simulink library "myLibrary"  (R2023b)
settings: Solver=VariableStepAuto  StartTime=0.0  StopTime=10.0  RelTol=1e-3
undefined symbols (not defined in the file): Cac_n1, ctrl1, Da, Discrete, dtha, ee_sli_rtmsupport, FA, gcbh, Ha, Ini, init_DCline, init_IPC, init_line, init_load, init_SG, init_shunt, init_TH, init_trafo, init_VSC, initMachineBlocks, Ka, Lf, Llkd_pu, Llkq1_pu, magnitude, NET, P, plots_step, q0, Rac_n1, Radd, Rkd_pu, Rkq1_pu, Rload_add, sim_config, sps_rtmsupport, spsSteamTurbineModel, T_DC_NET, T_global, T_IPC, T_load, T_NET, T_SG, T_shunt, T_STATCOM, T_TH, T_trafo, T_VSC, Ts, tstep, Udiff_a, V1
libraries: spsSeriesRLCBranchLib x105, eeGeneralControl x72, $bdroot x70, spsCurrentMeasurementLib x48, spsParallelRLCBranchLib x39, spsVoltageMeasurementLib x33, spsControlledVoltageSourceLib x27, spsFirstOrderFilterLib x16, dspsigops x6, spsThreePhaseVIMeasurementLib x5, spsPLL3phLib x4, spsThreePhaseBreakerLib x3
(part 1 of 12)
settings Model: Creator=CITCEA  LastModifiedBy=Josep
settings DebuggingCC: UnconnectedInputMsg=warning  UnconnectedOutputMsg=warning  UnconnectedLineMsg=warning
settings ModelReferenceCC: EnableRefExpFcnMdlSchedulingChecks=on
settings RTWCC: DLArmComputeVersion=19.05

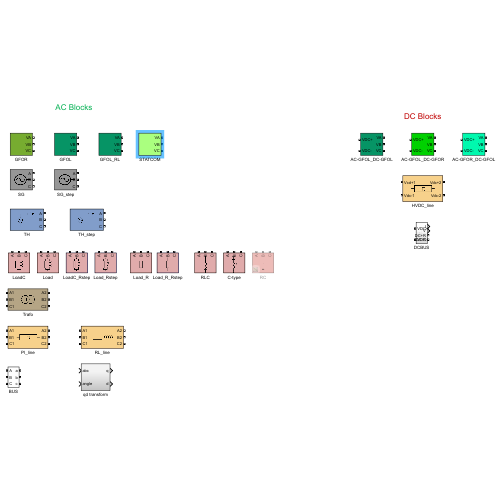
[thumbnail: Simulink's stored preview of the top-level diagram]
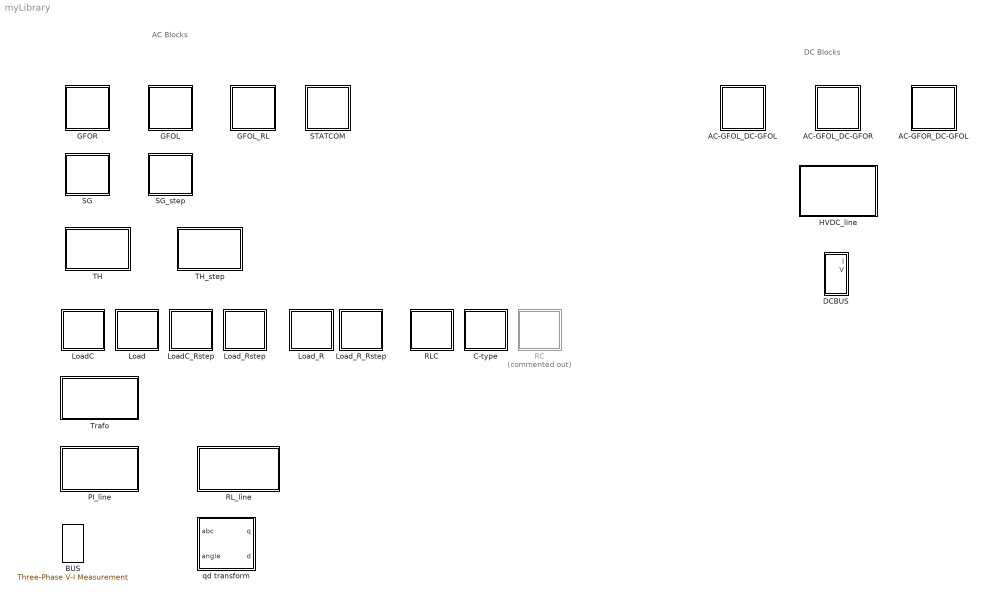
== system myLibrary ==
  note: DC Blocks
  note: AC Blocks
  AC-GFOL_DC-GFOL : Subsystem  mask{T_IPC_global=T_IPC, initIPC_global=init_IPC, num=1}
      mask prompts: T_IPC_global "T_IPC"; initIPC_global "init_IPC"
      mask init:
      | T_IPC = T_IPC_global(num,:);
      | initIPC = initIPC_global{num};
      | 
      | %set_param([gcb '/Control/Goto_w'],'GotoTag',['w_GFOL' num2str(num)])
      | %set_param([gcb '/Control/From_w'],'GotoTag',['w_GFOL' num2str(num)])
  AC-GFOL_DC-GFOR : Subsystem  mask{T_IPC_global=T_IPC, initIPC_global=init_IPC, num=1}
      mask prompts: T_IPC_global "T_IPC"; initIPC_global "init_IPC"
      mask init:
      | T_IPC = T_IPC_global(num,:);
      | initIPC = initIPC_global{num};
      | 
      | %set_param([gcb '/Control/Goto_w'],'GotoTag',['w_GFOL' num2str(num)])
      | %set_param([gcb '/Control/From_w'],'GotoTag',['w_GFOL' num2str(num)])
  AC-GFOR_DC-GFOL : Subsystem  mask{T_IPC_global=T_IPC, initIPC_global=init_IPC, num=1}
      mask prompts: T_IPC_global "T_IPC"; initIPC_global "init_IPC"
      mask init:
      | T_IPC = T_IPC_global(num,:);
      | initIPC = initIPC_global{num};
      | 
      | %set_param([gcb '/Control/Goto_w'],'GotoTag',['w_GFOL' num2str(num)])
      | %set_param([gcb '/Control/From_w'],'GotoTag',['w_GFOL' num2str(num)])
  BUS : spsThreePhaseVIMeasurementLib/Three-Phase V-I Measurement  VoltageMeasurement=phase-to-phase  SetLabelV=on  LabelV=V  Vpu=off  VpuLL=off  CurrentMeasurement=yes  SetLabelI=on  LabelI=I  Ipu=off  Pbase=100e6  Vbase=500e3  OutputType=Complex  PhasorSimulation=off  PSBequivalent=0
  C-type : Subsystem  mask{T_shunt_global=T_shunt, initShunt_global=init_shunt, num=1}
      mask prompts: T_shunt_global "T_shunt"; initShunt_global "init_shunt"
      mask init:
      | T = T_shunt_global(num,:);
      | ini = initShunt_global{num};
      mask Display:
      | % Use specified image as mask icon
      | image('C-type.png')
  DCBUS : Subsystem
  GFOL : Subsystem  mask{T_VSC_global=T_VSC, initVSC_global=init_VSC, num=1}
      mask prompts: T_VSC_global "T_VSC"; initVSC_global "init_VSC"
      mask init:
      | T_VSC = T_VSC_global(num,:);
      | initVSC = initVSC_global{num};
      | 
      | set_param([gcb '/Control/Goto_w'],'GotoTag',['w_GFOL' num2str(num)])
      | set_param([gcb '/Control/From_w'],'GotoTag',['w_GFOL' num2str(num)])
  GFOL_RL : Subsystem  mask{T_VSC_global=T_VSC, initVSC_global=init_VSC, num=1}
      mask prompts: T_VSC_global "T_VSC"; initVSC_global "init_VSC"
      mask init:
      | T_VSC = T_VSC_global(num,:);
      | initVSC = initVSC_global{num};
      | 
      | set_param([gcb '/Control/Goto_w'],'GotoTag',['w_GFOL' num2str(num)])
      | set_param([gcb '/Control/From_w'],'GotoTag',['w_GFOL' num2str(num)])
  GFOR : Subsystem  mask{T_VSC_global=T_VSC, initVSC_global=init_VSC, num=1}
      mask prompts: T_VSC_global "T_VSC"; initVSC_global "init_VSC"
      mask init:
      | T_VSC = T_VSC_global(num,:);
      | initVSC = initVSC_global{num};
      | 
      | set_param([gcb '/Control/Goto_theta'],'GotoTag',['theta_GFOR' num2str(num)])
      | set_param([gcb '/Control/PLL/Goto_w'],'GotoTag',['w_GFOR' num2str(num)])
  HVDC_line : Subsystem  mask{T_HVDC_line_global=T_DC_NET, initDCLine_global=init_DCline, num=1}
      mask prompts: T_HVDC_line_global "T_DC_line"; initDCLine_global "init_DCline"
      mask init:
      | T = T_HVDC_line_global(num,:);
      | ini = initDCLine_global{num};
      mask Display:
      | % Use specified image as mask icon
      | image('PI.png')
  Load : Subsystem  mask{T_load_global=T_load, initLoad_global=init_load, num=1}
      mask prompts: T_load_global "T_load"; initLoad_global "init_load"
      mask init:
      | T = T_load_global(num,:);
      | ini = initLoad_global{num};
      mask Display:
      | % Use specified image as mask icon
      | image('load.png')
  LoadC : Subsystem  mask{T_load_global=T_load, initLoad_global=init_load, num=1}
      mask prompts: T_load_global "T_load"; initLoad_global "init_load"
      mask init:
      | T = T_load_global(num,:);
      | ini = initLoad_global{num};
      mask Display:
      | % Use specified image as mask icon
      | image('load.png')
  LoadC_Rstep : Subsystem  mask{T_load_global=T_load, initLoad_global=init_load, num=1, tstep=tstep, Radd=Radd}
      mask prompts: T_load_global "T_load"; initLoad_global "init_load"
      mask init:
      | T = T_load_global(num,:);
      | ini = initLoad_global{num};
      mask Display:
      | % Use specified image as mask icon
      | image('load.png')
  Load_R : Subsystem  mask{T_load_global=T_load, num=1}
      mask prompts: T_load_global "T_load"
      mask init:
      | T = T_load_global(num,:);
      mask Display:
      | % Use specified image as mask icon
      | image('load_R.png')
  Load_R_Rstep : Subsystem  mask{T_load_global=T_load, num=1, tstep=tstep, Radd=Radd}
      mask prompts: T_load_global "T_load"
      mask init:
      | T = T_load_global(num,:);
      mask Display:
      | % Use specified image as mask icon
      | image('load_R.png')
  Load_Rstep : Subsystem  mask{T_load_global=T_load, initLoad_global=init_load, num=1, tstep=tstep, Radd=Radd}
      mask prompts: T_load_global "T_load"; initLoad_global "init_load"
      mask init:
      | T = T_load_global(num,:);
      | ini = initLoad_global{num};
      mask Display:
      | % Use specified image as mask icon
      | image('load.png')
  PI_line : Subsystem  mask{T_line_global=T_NET, initLine_global=init_line, num=1, set_C0=ones(1,6), set_iL0=0}
      mask prompts: T_line_global "T_line"; initLine_global "init_line"; set_C0 "init_cap"; set_iL0 "init_ind"
      mask init:
      | T = T_line_global(num,:);
      | ini = initLine_global{num};
      | set_C00 = set_C0(1,1);
      | set_C01 = set_C0(1,2);
      | set_C02 = set_C0(1,3);
      | set_C03 = set_C0(1,4);
      | set_C04 = set_C0(1,5);
      | set_C05 = set_C0(1,6);
      | set_param([gcb '/Series RLC Branch'],'Setx0',set_C00)
      | set_param([gcb '/Series RLC Branch1'],'Setx0',set_C01)
      | set_param([gcb '/Series RLC Branch2'],'Setx0',set_C02)
      | set_param([gcb '/Series RLC Branch3'],'Setx0',set_C03)
      | set_param([gcb '/Series RLC Branch4'],'Setx0',set_C04)
      | set_param([gcb '/Series RLC Branch5'],'Setx0',set_C05)
      | set_param([gcb '/Series RLC Branch6'],'SetiL0',set_iL0)
      mask Display:
      | % Use specified image as mask icon
      | image('PI.png')
  RC : Subsystem  Commented=on  mask{T_shunt_global=T_shunt, initShunt_global=init_shunt, num=1}
      mask prompts: T_shunt_global "T_shunt"; initShunt_global "init_shunt"
      mask init:
      | T = T_shunt_global(num,:);
      | ini = initShunt_global{num};
      mask Display:
      | % Use specified image as mask icon
      | image('RC.png')
  RLC : Subsystem  mask{T_shunt_global=T_shunt, initShunt_global=init_shunt, num=1}
      mask prompts: T_shunt_global "T_shunt"; initShunt_global "init_shunt"
      mask init:
      | T = T_shunt_global(num,:);
      | ini = initShunt_global{num};
      mask Display:
      | % Use specified image as mask icon
      | image('RLC.png')
  RL_line : Subsystem  mask{T_line_global=T_NET, initLine_global=init_line, num=1}
      mask prompts: T_line_global "T_line"; initLine_global "init_line"
      mask init:
      | T = T_line_global(num,:);
      | ini = initLine_global{num};
      mask Display:
      | % Use specified image as mask icon
      | image('RL.png')
  SG : Subsystem  mask{num=1, init_SG_global=init_SG, initMachineBlocks=initMachineBlocks, T_SG_global=T_SG}
      mask prompts: init_SG_global "init_SG"; initMachineBlocks "initMachine"; T_SG_global "T_SG"
      mask init:
      | initSG = init_SG_global{num};
      | T_SG = T_SG_global(num,:);
      | SGnum = num;
      | 
      | T_SG.exc = T_SG.exc{:};
      | T_SG.mech = T_SG.mech{:};
      | T_SG.PSS = T_SG.PSS{:};
      | 
      | 
      | switch T_SG.pss{:}
      |     case '2A'
      |         hasPSS = 1;
      |         set_param([gcb '/Exciter/PSS 2A'],'commented', 'off')
      |     case 'no'
      |         hasPSS = 0;
      |         set_param([gcb '/Exciter/PSS 2A'],'commented', 'on')
      | end
      | 
      | switch T_SG.govturb{:}
      |     case 'IEEEG1'
      |         selectGovturb= 1;
      |         set_param([gcb '/Governor-Turbine/IEEEG1'],'commented', 'off')
      |         set_param([gcb '/Governor-Turbine/Steam Turbine and Governor'],'commented', 'on')
      |     case 'TANDEM-SINGLE'
      |         selectGovturb= 2;
      |         T_SG.genType = 0;
      |         set_param([gcb '/Governor-Turbine/IEEEG1'],'commented', 'on')
      |         set_param([gcb '/Governor-Turbine/Steam Turbine and Governor'],'commented', 'off')
      |     case 'TANDEM-MULTI'
      |         selectGovturb= 2;
      |         T_SG.genType = 1;
      |         set_param([gcb '/Governor-Turbine/IEEEG1'],'commented', 'on')
      |         set_param([gcb '/Governor-Turbine/Steam Turbine and Governor'],'commented', 'off')
      |     case 'no'
      |         selectGovturb= 3;
      |         set_param([gcb '/Governor-Turbine/IEEEG1'],'commented', 'on')
      |         set_param([gcb '/Governor-Turbine/Steam Turbine and Governor'],'commented', 'on')
      | end
      | 
      | switch T_SG.exciter{:} 
      |     case 'AC4A'
      |         selectExciter = 1;
      |         set_param([gcb '/Exciter/Exciter AC4A'],'commented', 'off')
      |         set_param([gcb '/Exciter/Exciter ST4B'],'commented', 'on')
      |         set_param([gcb '/Exciter/Exciter ST1'],'commented', 'on')
      |     case 'ST4B'
      |         selectExciter = 2;
      |         set_param([gcb '/Exciter/Exciter AC4A'],'commented', 'on')
      |         set_param([gcb '/Exciter/Exciter ST4B'],'commented', 'off')
      |         set_param([gcb '/Exciter/Exciter ST1'],'commented', 'on')
      |     case 'ST1'
      |         selectExciter = 3;
      |         set_param([gcb '/Exciter/Exciter AC4A'],'commented', 'on')
      |         set_param([gcb '/Exciter/Exciter ST4B'],'commented', 'on')
      |         set_param([gcb '/Exciter/Exciter ST1'],'commented', 'off')
      |     case 'no'
      |         selectExciter = 4;
      |         set_param([gcb '/Exciter/Exciter AC4A'],'commented', 'on')
      |         set_param([gcb '/Exciter/Exciter ST4B'],'commented', 'on')
      |         set_param([gcb '/Exciter/Exciter ST1'],'commented', 'on')
      | end
      | 
      | set_param([gcb '/Goto_theta'],'GotoTag',['theta_SG' num2str(SGnum)])
      | set_param([gcb '/Goto_w'],'GotoTag',['w_SG' num2str(SGnum)])
      mask Display:
      | % Use specified image as mask icon
      | image('SG.png')
  SG_step : Subsystem  mask{num=1, init_SG_global=init_SG, initMachineBlocks=initMachineBlocks, T_SG_global=T_SG, step_var=Pref, tstep=sim_config.tstep}
      mask prompts: init_SG_global "init_SG"; initMachineBlocks "initMachine"; T_SG_global "T_SG"
      mask init:
      | initSG = init_SG_global{num};
      | T_SG = T_SG_global(num,:);
      | SGnum = num;
      | 
      | T_SG.exc = T_SG.exc{:};
      | T_SG.mech = T_SG.mech{:};
      | T_SG.PSS = T_SG.PSS{:};
      | 
      | 
      | switch T_SG.pss{:}
      |     case '2A'
      |         hasPSS = 1;
      |         set_param([gcb '/Exciter/PSS 2A'],'commented', 'off')
      |     case 'no'
      |         hasPSS = 0;
      |         set_param([gcb '/Exciter/PSS 2A'],'commented', 'on')
      | end
      | 
      | switch T_SG.govturb{:}
      |     case 'IEEEG1'
      |         selectGovturb= 1;
      |         set_param([gcb '/Governor-Turbine/IEEEG1'],'commented', 'off')
      |         set_param([gcb '/Governor-Turbine/Steam Turbine and Governor'],'commented', 'on')
      |     case 'TANDEM-SINGLE'
      |         selectGovturb= 2;
      |         T_SG.genType = 0;
      |         set_param([gcb '/Governor-Turbine/IEEEG1'],'commented', 'on')
      |         set_param([gcb '/Governor-Turbine/Steam Turbine and Governor'],'commented', 'off')
      |     case 'TANDEM-MULTI'
      |         selectGovturb= 2;
      |         T_SG.genType = 1;
      |         set_param([gcb '/Governor-Turbine/IEEEG1'],'commented', 'on')
      |         set_param([gcb '/Governor-Turbine/Steam Turbine and Governor'],'commented', 'off')
      |     case 'no'
      |         selectGovturb= 3;
      |         set_param([gcb '/Governor-Turbine/IEEEG1'],'commented', 'on')
      |         set_param([gcb '/Governor-Turbine/Steam Turbine and Governor'],'commented', 'on')
      | end
      | 
      | switch T_SG.exciter{:} 
      |     case 'AC4A'
      |         selectExciter = 1;
      |         set_param([gcb '/Exciter/Exciter AC4A'],'commented', 'off')
      |         set_param([gcb '/Exciter/Exciter ST4B'],'commented', 'on')
      |         set_param([gcb '/Exciter/Exciter ST1'],'commented', 'on')
      |     case 'ST4B'
      |         selectExciter = 2;
      |         set_param([gcb '/Exciter/Exciter AC4A'],'commented', 'on')
      |         set_param([gcb '/Exciter/Exciter ST4B'],'commented', 'off')
      |         set_param([gcb '/Exciter/Exciter ST1'],'commented', 'on')
      |     case 'ST1'
      |         selectExciter = 3;
      |         set_param([gcb '/Exciter/Exciter AC4A'],'commented', 'on')
      |         set_param([gcb '/Exciter/Exciter ST4B'],'commented', 'on')
      |         set_param([gcb '/Exciter/Exciter ST1'],'commented', 'off')
      |     case 'no'
      |         selectExciter = 4;
      |         set_param([gcb '/Exciter/Exciter AC4A'],'commented', 'on')
      |         set_param([gcb '/Exciter/Exciter ST4B'],'commented', 'on')
      |         set_param([gcb '/Exciter/Exciter ST1'],'commented', 'on')
      | end
      | 
      | set_param([gcb '/Goto_theta'],'GotoTag',['theta_SG' num2str(SGnum)])
      | set_param([gcb '/Goto_w'],'GotoTag',['w_SG' num2str(SGnum)])
      | 
      | switch step_var
      |     case 'Pref'
      |         tstep_P = tstep;
      |         tstep_V = 1e3;
      |     case 'Vref'
      |         tstep_P = 1e3;
      |         tstep_V = tstep;
      | end
      mask TypeOptions step_var: Pref | Vref
      mask Display:
      | % Use specified image as mask icon
      | image('SG.png')
  STATCOM : Subsystem  mask{T_VSC_global=T_VSC, initVSC_global=init_VSC, num=1}
      mask prompts: T_VSC_global "T_VSC"; initVSC_global "init_VSC"
      mask init:
      | T_VSC = T_VSC_global(num,:);
      | initVSC = initVSC_global{num};
      | 
      | switch T_VSC.POD{:}
      |     case 'Yes'
      |         POD = 1;
      |         set_param([gcb '/Control/POD'],'commented', 'off')
      |         set_param([gcb '/Control/From34'],'commented', 'off')
      |         set_param([gcb '/Control/From35'],'commented', 'off')
      |         set_param([gcb '/Control/From36'],'commented', 'off')
      |         set_param([gcb '/Control/From37'],'commented', 'off')
      |     case 'No'
      |         POD = 2;
      |         set_param([gcb '/Control/POD'],'commented', 'on')
      |         set_param([gcb '/Control/From34'],'commented', 'on')
      |         set_param([gcb '/Control/From35'],'commented', 'on')
      |         set_param([gcb '/Control/From36'],'commented', 'on')
      |         set_param([gcb '/Control/From37'],'commented', 'on')
      | end
      | 
      | 
      | 
      | set_param([gcb '/Control/Goto_w'],'GotoTag',['w_STATCOM' num2str(num)])
  TH : Subsystem  mask{T_TH_global=T_TH, initTH_global=init_TH, num=1}
      mask prompts: T_TH_global "T_TH"; initTH_global "init_TH"
      mask init:
      | T = T_TH_global(num,:);
      | ini = initTH_global{num};
      mask Display:
      | port_label('rconn', 1, 'A')
      | port_label('rconn', 2, 'B')
      | port_label('rconn', 3, 'C')
      | 
      | % Use specified image as mask icon
      | image('TH.png')
  TH_step : Subsystem  mask{T_TH_global=T_TH, initTH_global=init_TH, num=1, tstep=tstep, V1=V1}
      mask prompts: T_TH_global "T_TH"; initTH_global "init_TH"
      mask init:
      | T = T_TH_global(num,:);
      | ini = initTH_global{num};
      mask Display:
      | port_label('rconn', 1, 'A')
      | port_label('rconn', 2, 'B')
      | port_label('rconn', 3, 'C')
      | 
      | % Use specified image as mask icon
      | image('TH.png')
  Trafo : Subsystem  mask{T_trafo_global=T_trafo, initTrafo_global=init_trafo, num=3}
      mask prompts: T_trafo_global "T_trafo"; initTrafo_global "init_trafo"
      mask init:
      | T = T_trafo_global(num,:);
      | ini = initTrafo_global{num};
      mask Display:
      | % Use specified image as mask icon
      | image('trafo.png')
  qd transform : Subsystem

== system myLibrary/AC-GFOL_DC-GFOL ==
  Constant1 : Constant  Value=[ 2/3 1/3; -1/3 1/3 ; -1/3 -2/3]
  Control Pac2 : Subsystem
      settings: PortSchema="{\"entries\":[{\"content\":{\"sides\":[{\"content\":{},\"type\":\"ConnectorPlacement.EquallySpacedRectSide\",\"uuid\":\"681c0b5f-022d-4b6d-8fe2-73940743a76e\"},{\"content\":{\"side\":\"RIGHT\"},\"type\":\"ConnectorPlacement.EquallySpacedRectSide\",\"uuid\":\"e9b400c8-e13f-4caf-91a1-f348979675fd\"},{\"content\":{\"connectorIds\":[\"Out1\"],\"side\":\"TOP\"},\"type\":\"ConnectorPlacement.EquallySpacedRectSide\",\"uuid\":\"348007cb-ce67-4c45-ad7b-36ba89db6185\"},{\"content\":{\"connectorIds\":[\"In1\",\"In2\",\"In3\",\"In4\",\"In5\",\"In6\"],\"side\":\"BOTTOM\"},\"type\":\"ConnectorPlacement.EquallySpacedRectSide\",\"uuid\":\"fd6a847a-5d69-44cd-a0d1-495126761350\"}]},\"type\":\"ConnectorPlacement.EquallySpacedConnector\",\"uuid\":\"d16b8cae-5ced-4c76-a87e-983e154fb48f\"}],\"packageUris\":[\"http://schema.mathworks.com/mf0/Connector/R2020b\"],\"version\":\"1.0\"}"
  Is_l2g1 : Gain  Gain=1/T_IPC.Ibpu_l2g
  Is_l2g2 : Gain  Gain=1/T_IPC.Ibpu_l2g
  Is_l2g3 : Gain  Gain=1/T_IPC.Ibpu_l2g
  MMC1 : Subsystem
  Mesura Ulina12 : spsVoltageMeasurementLib/Voltage Measurement  PhasorSimulation=off  OutputType=Complex  PSBequivalent=0
  Mux1 : Mux  Inputs=2
  Product1 : Product  Multiplication=Matrix(*)
  Scope : Scope
  Scope1 : Scope
  U_g2l1 : Gain  Gain=1/T_IPC.Vbpu_l2g
  U_g2l2 : Gain  Gain=1/T_IPC.Vbpu_l2g
  U_g2l3 : Gain  Gain=1/T_IPC.Vbpu_l2g
  Vdiff_l2g1 : Gain  Gain=T_IPC.Vbpu_l2g
  Voltage Measurement2 : spsVoltageMeasurementLib/Voltage Measurement  PhasorSimulation=off  OutputType=Complex  PSBequivalent=0
  Voltage Measurement3 : spsVoltageMeasurementLib/Voltage Measurement  PhasorSimulation=off  OutputType=Complex  PSBequivalent=0
  VA : PMIOPort  Side=Right
  VB : PMIOPort  Port=2  Side=Right
  VC : PMIOPort  Port=3  Side=Right
  VDC+ : PMIOPort  Port=4  Side=Left
  VDC- : PMIOPort  Port=5  Side=Left
  wires:
  Voltage Measurement3/1 -> Mux1/2
  Mux1/1 -> Product1/2
  Constant1/1 -> Product1/1
  MMC1/4(Vs) -> U_g2l2/1
  Product1/1 -> Scope1/1, U_g2l1/1
  Control Pac2/1(Vdiff-sum) -> Vdiff_l2g1/1
  Mesura Ulina12/1 -> U_g2l3/1, Scope/1
  MMC1/2(Iu) -> Is_l2g2/1
  MMC1/1(Is) -> Is_l2g3/1
  MMC1/3(Il) -> Is_l2g1/1
  Voltage Measurement2/1 -> Mux1/1
  Vdiff_l2g1/1 -> MMC1/1(Vdiff,sum)
  U_g2l1/1 -> Control Pac2/1(U)
  U_g2l2/1 -> Control Pac2/3(Vs)
  U_g2l3/1 -> Control Pac2/2(Vdc2)
  Is_l2g1/1 -> Control Pac2/4(Il)
  Is_l2g2/1 -> Control Pac2/5(Iu)
  Is_l2g3/1 -> Control Pac2/6(Iss)
  connections:
  Voltage Measurement3/LConn1 -- MMC1/LConn2 -- Voltage Measurement2/LConn2 -- VB/RConn1
  VDC-/RConn1 -- MMC1/RConn2 -- Mesura Ulina12/LConn2
  Voltage Measurement2/LConn1 -- MMC1/LConn1 -- VA/RConn1
  VDC+/RConn1 -- MMC1/RConn1 -- Mesura Ulina12/LConn1
  VC/RConn1 -- MMC1/LConn3 -- Voltage Measurement3/LConn2

== system myLibrary/AC-GFOL_DC-GFOR ==
  Constant1 : Constant  Value=[ 2/3 1/3; -1/3 1/3 ; -1/3 -2/3]
  Control Pac2 : Subsystem
      settings: PortSchema="{\"entries\":[{\"content\":{\"sides\":[{\"content\":{},\"type\":\"ConnectorPlacement.EquallySpacedRectSide\",\"uuid\":\"681c0b5f-022d-4b6d-8fe2-73940743a76e\"},{\"content\":{\"side\":\"RIGHT\"},\"type\":\"ConnectorPlacement.EquallySpacedRectSide\",\"uuid\":\"e9b400c8-e13f-4caf-91a1-f348979675fd\"},{\"content\":{\"connectorIds\":[\"Out1\"],\"side\":\"TOP\"},\"type\":\"ConnectorPlacement.EquallySpacedRectSide\",\"uuid\":\"348007cb-ce67-4c45-ad7b-36ba89db6185\"},{\"content\":{\"connectorIds\":[\"In1\",\"In2\",\"In3\",\"In4\",\"In5\",\"In6\"],\"side\":\"BOTTOM\"},\"type\":\"ConnectorPlacement.EquallySpacedRectSide\",\"uuid\":\"fd6a847a-5d69-44cd-a0d1-495126761350\"}]},\"type\":\"ConnectorPlacement.EquallySpacedConnector\",\"uuid\":\"d16b8cae-5ced-4c76-a87e-983e154fb48f\"}],\"packageUris\":[\"http://schema.mathworks.com/mf0/Connector/R2020b\"],\"version\":\"1.0\"}"
  Is_l2g1 : Gain  Gain=1/T_IPC.Ibpu_l2g
  Is_l2g2 : Gain  Gain=1/T_IPC.Ibpu_l2g
  Is_l2g3 : Gain  Gain=1/T_IPC.Ibpu_l2g
  MMC1 : Subsystem
  Mesura Ulina12 : spsVoltageMeasurementLib/Voltage Measurement  PhasorSimulation=off  OutputType=Complex  PSBequivalent=0
  Mux1 : Mux  Inputs=2
  Product1 : Product  Multiplication=Matrix(*)
  Scope : Scope
  Scope1 : Scope
  U_g2l1 : Gain  Gain=1/T_IPC.Vbpu_l2g
  U_g2l2 : Gain  Gain=1/T_IPC.Vbpu_l2g
  U_g2l3 : Gain  Gain=1/T_IPC.Vbpu_l2g
  Vdiff_l2g1 : Gain  Gain=T_IPC.Vbpu_l2g
  Voltage Measurement2 : spsVoltageMeasurementLib/Voltage Measurement  PhasorSimulation=off  OutputType=Complex  PSBequivalent=0
  Voltage Measurement3 : spsVoltageMeasurementLib/Voltage Measurement  PhasorSimulation=off  OutputType=Complex  PSBequivalent=0
  VA : PMIOPort  Side=Right
  VB : PMIOPort  Port=2  Side=Right
  VC : PMIOPort  Port=3  Side=Right
  VDC+ : PMIOPort  Port=4  Side=Left
  VDC- : PMIOPort  Port=5  Side=Left
  wires:
  Voltage Measurement3/1 -> Mux1/2
  Mux1/1 -> Product1/2
  Constant1/1 -> Product1/1
  MMC1/4(Vs) -> U_g2l2/1
  Product1/1 -> Scope1/1, U_g2l1/1
  Control Pac2/1(Vdiff-sum) -> Vdiff_l2g1/1
  Mesura Ulina12/1 -> U_g2l3/1, Scope/1
  MMC1/2(Iu) -> Is_l2g2/1
  MMC1/1(Is) -> Is_l2g3/1
  MMC1/3(Il) -> Is_l2g1/1
  Voltage Measurement2/1 -> Mux1/1
  Vdiff_l2g1/1 -> MMC1/1(Vdiff,sum)
  U_g2l1/1 -> Control Pac2/1(U)
  U_g2l2/1 -> Control Pac2/3(Vs)
  U_g2l3/1 -> Control Pac2/2(Vdc)
  Is_l2g1/1 -> Control Pac2/4(Il)
  Is_l2g2/1 -> Control Pac2/5(Iu)
  Is_l2g3/1 -> Control Pac2/6(Iss)
  connections:
  MMC1/LConn2 -- Voltage Measurement3/LConn1 -- Voltage Measurement2/LConn2 -- VB/RConn1
  MMC1/RConn2 -- VDC-/RConn1 -- Mesura Ulina12/LConn2
  MMC1/LConn1 -- Voltage Measurement2/LConn1 -- VA/RConn1
  VDC+/RConn1 -- Mesura Ulina12/LConn1 -- MMC1/RConn1
  MMC1/LConn3 -- VC/RConn1 -- Voltage Measurement3/LConn2

== system myLibrary/AC-GFOR_DC-GFOL ==
  Constant1 : Constant  Value=[ 2/3 1/3; -1/3 1/3 ; -1/3 -2/3]
  Control Pac2 : Subsystem
      settings: PortSchema="{\"entries\":[{\"content\":{\"sides\":[{\"content\":{},\"type\":\"ConnectorPlacement.EquallySpacedRectSide\",\"uuid\":\"681c0b5f-022d-4b6d-8fe2-73940743a76e\"},{\"content\":{\"side\":\"RIGHT\"},\"type\":\"ConnectorPlacement.EquallySpacedRectSide\",\"uuid\":\"e9b400c8-e13f-4caf-91a1-f348979675fd\"},{\"content\":{\"connectorIds\":[\"Out1\"],\"side\":\"TOP\"},\"type\":\"ConnectorPlacement.EquallySpacedRectSide\",\"uuid\":\"348007cb-ce67-4c45-ad7b-36ba89db6185\"},{\"content\":{\"connectorIds\":[\"In1\",\"In2\",\"In3\",\"In4\",\"In5\",\"In6\"],\"side\":\"BOTTOM\"},\"type\":\"ConnectorPlacement.EquallySpacedRectSide\",\"uuid\":\"fd6a847a-5d69-44cd-a0d1-495126761350\"}]},\"type\":\"ConnectorPlacement.EquallySpacedConnector\",\"uuid\":\"d16b8cae-5ced-4c76-a87e-983e154fb48f\"}],\"packageUris\":[\"http://schema.mathworks.com/mf0/Connector/R2020b\"],\"version\":\"1.0\"}"
  Is_l2g1 : Gain  Gain=1/T_IPC.Ibpu_l2g
  Is_l2g2 : Gain  Gain=1/T_IPC.Ibpu_l2g
  Is_l2g3 : Gain  Gain=1/T_IPC.Ibpu_l2g
  MMC1 : Subsystem
  Mesura Ulina12 : spsVoltageMeasurementLib/Voltage Measurement  PhasorSimulation=off  OutputType=Complex  PSBequivalent=0
  Mux1 : Mux  Inputs=2
  Product1 : Product  Multiplication=Matrix(*)
  Scope : Scope
  U_g2l1 : Gain  Gain=1/T_IPC.Vbpu_l2g
  U_g2l2 : Gain  Gain=1/T_IPC.Vbpu_l2g
  U_g2l3 : Gain  Gain=1/T_IPC.Vbpu_l2g
  Vdiff_l2g1 : Gain  Gain=T_IPC.Vbpu_l2g
  Voltage Measurement2 : spsVoltageMeasurementLib/Voltage Measurement  PhasorSimulation=off  OutputType=Complex  PSBequivalent=0
  Voltage Measurement3 : spsVoltageMeasurementLib/Voltage Measurement  PhasorSimulation=off  OutputType=Complex  PSBequivalent=0
  VA : PMIOPort  Side=Right
  VB : PMIOPort  Port=2  Side=Right
  VC : PMIOPort  Port=3  Side=Right
  VDC+ : PMIOPort  Port=4  Side=Left
  VDC- : PMIOPort  Port=5  Side=Left
  wires:
  Is_l2g3/1 -> Control Pac2/6(Iss)
  Is_l2g2/1 -> Control Pac2/5(Iu)
  Is_l2g1/1 -> Control Pac2/4(Il)
  U_g2l3/1 -> Control Pac2/2(Vdc)
  U_g2l2/1 -> Control Pac2/3(Vs)
  U_g2l1/1 -> Control Pac2/1(U)
  Vdiff_l2g1/1 -> MMC1/1(Vdiff,sum)
  Voltage Measurement2/1 -> Mux1/1
  MMC1/3(Il) -> Is_l2g1/1
  MMC1/1(Is) -> Is_l2g3/1
  MMC1/2(Iu) -> Is_l2g2/1
  Mesura Ulina12/1 -> Scope/1, U_g2l3/1
  Control Pac2/1(Vdiff-sum) -> Vdiff_l2g1/1
  Product1/1 -> U_g2l1/1
  MMC1/4(Vs) -> U_g2l2/1
  Constant1/1 -> Product1/1
  Mux1/1 -> Product1/2
  Voltage Measurement3/1 -> Mux1/2
  connections:
  Voltage Measurement3/LConn2 -- VC/RConn1 -- MMC1/LConn3
  MMC1/RConn1 -- Mesura Ulina12/LConn1 -- VDC+/RConn1
  VA/RConn1 -- Voltage Measurement2/LConn1 -- MMC1/LConn1
  Mesura Ulina12/LConn2 -- VDC-/RConn1 -- MMC1/RConn2
  VB/RConn1 -- Voltage Measurement2/LConn2 -- Voltage Measurement3/LConn1 -- MMC1/LConn2

== system myLibrary/C-type ==
  C1a : spsSeriesRLCBranchLib/Series RLC Branch  LConnTagsString=__new0  RConnTagsString=__new0  BranchType=C  Resistance=T_STATCOM.Rshunt  Inductance=T_STATCOM.Lshunt  SetiL0=off  InitialCurrent=initMMC.iL_a  Capacitance=T.C1*T.Zbpu_l2g  Setx0=on  InitialVoltage=ini.vC1_a  Measurements=Branch voltage
  C1b : spsSeriesRLCBranchLib/Series RLC Branch  LConnTagsString=__new0  RConnTagsString=__new0  BranchType=C  Resistance=T_STATCOM.Rshunt  Inductance=T_STATCOM.Lshunt  SetiL0=off  InitialCurrent=initMMC.iL_a  Capacitance=T.C1*T.Zbpu_l2g  Setx0=on  InitialVoltage=ini.vC1_b  Measurements=Branch voltage
  C1c : spsSeriesRLCBranchLib/Series RLC Branch  LConnTagsString=__new0  RConnTagsString=__new0  BranchType=C  Resistance=T_STATCOM.Rshunt  Inductance=T_STATCOM.Lshunt  SetiL0=off  InitialCurrent=initMMC.iL_a  Capacitance=T.C1*T.Zbpu_l2g  Setx0=on  InitialVoltage=ini.vC1_c  Measurements=Branch voltage
  C2a : spsSeriesRLCBranchLib/Series RLC Branch  LConnTagsString=__new0  RConnTagsString=__new0  BranchType=C  Resistance=T_STATCOM.Rshunt  Inductance=T_STATCOM.L_ctype  SetiL0=on  InitialCurrent=initMMC.iL_ctype_a  Capacitance=T.C2*T.Zbpu_l2g  Setx0=on  InitialVoltage=ini.vC2_a  Measurements=Branch voltage
  C2b : spsSeriesRLCBranchLib/Series RLC Branch  LConnTagsString=__new0  RConnTagsString=__new0  BranchType=C  Resistance=T_STATCOM.Rshunt  Inductance=T_STATCOM.L_ctype  SetiL0=on  InitialCurrent=initMMC.iL_ctype_b  Capacitance=T.C2*T.Zbpu_l2g  Setx0=on  InitialVoltage=ini.vC2_b  Measurements=Branch voltage
  C2c : spsSeriesRLCBranchLib/Series RLC Branch  LConnTagsString=__new0  RConnTagsString=__new0  BranchType=C  Resistance=T_STATCOM.Rshunt  Inductance=T_STATCOM.L_ctype  SetiL0=on  InitialCurrent=initMMC.iL_ctype_c  Capacitance=T.C2*T.Zbpu_l2g  Setx0=on  InitialVoltage=ini.vC2_c  Measurements=Branch voltage
  La : spsSeriesRLCBranchLib/Series RLC Branch  LConnTagsString=__new0  RConnTagsString=__new0  BranchType=L  Resistance=T_STATCOM.Rshunt  Inductance=T.L/T.Zbpu_l2g  SetiL0=on  InitialCurrent=ini.iL_a  Capacitance=T_STATCOM.C2_ctype  Setx0=on  InitialVoltage=initMMC.vc2_a  Measurements=Branch current
  Lb : spsSeriesRLCBranchLib/Series RLC Branch  LConnTagsString=__new0  RConnTagsString=__new0  BranchType=L  Resistance=T_STATCOM.Rshunt  Inductance=T.L/T.Zbpu_l2g  SetiL0=on  InitialCurrent=ini.iL_b  Capacitance=T_STATCOM.C2_ctype  Setx0=on  InitialVoltage=initMMC.vc2_b  Measurements=Branch current
  Lc : spsSeriesRLCBranchLib/Series RLC Branch  LConnTagsString=__new0  RConnTagsString=__new0  BranchType=L  Resistance=T_STATCOM.Rshunt  Inductance=T.L/T.Zbpu_l2g  SetiL0=on  InitialCurrent=ini.iL_c  Capacitance=T_STATCOM.C2_ctype  Setx0=on  InitialVoltage=initMMC.vc2_c  Measurements=Branch current
  Ra : spsSeriesRLCBranchLib/Series RLC Branch  LConnTagsString=__new0  RConnTagsString=__new0  BranchType=R  Resistance=T.R/T.Zbpu_l2g  Inductance=T_STATCOM.Lshunt  SetiL0=off  InitialCurrent=initMMC.iL_a  Capacitance=T_STATCOM.Cshunt  Setx0=off  InitialVoltage=initMMC.vc_a  Measurements=None
  Rb : spsSeriesRLCBranchLib/Series RLC Branch  LConnTagsString=__new0  RConnTagsString=__new0  BranchType=R  Resistance=T.R/T.Zbpu_l2g  Inductance=T_STATCOM.Lshunt  SetiL0=off  InitialCurrent=initMMC.iL_a  Capacitance=T_STATCOM.Cshunt  Setx0=off  InitialVoltage=initMMC.vc_a  Measurements=None
  Rc : spsSeriesRLCBranchLib/Series RLC Branch  LConnTagsString=__new0  RConnTagsString=__new0  BranchType=R  Resistance=T.R/T.Zbpu_l2g  Inductance=T_STATCOM.Lshunt  SetiL0=off  InitialCurrent=initMMC.iL_a  Capacitance=T_STATCOM.Cshunt  Setx0=off  InitialVoltage=initMMC.vc_a  Measurements=None
  A : PMIOPort  Side=Left
  B : PMIOPort  Port=2  Side=Left
  C : PMIOPort  Port=3  Side=Left
  connections:
  C1c/LConn1 -- C/RConn1
  C1b/LConn1 -- B/RConn1
  C1a/LConn1 -- A/RConn1
  C2c/RConn1 -- Rb/RConn1 -- C2a/RConn1 -- Ra/RConn1 -- C2b/RConn1 -- Rc/RConn1
  Rc/LConn1 -- C1c/RConn1 -- Lc/LConn1
  Ra/LConn1 -- C1a/RConn1 -- La/LConn1
  Rb/LConn1 -- Lb/LConn1 -- C1b/RConn1
  C2c/LConn1 -- Lc/RConn1
  C2a/LConn1 -- La/RConn1
  C2b/LConn1 -- Lb/RConn1

== system myLibrary/DCBUS ==
  Current Measurement : spsCurrentMeasurementLib/Current Measurement  PhasorSimulation=off  OutputType=Complex  PSBequivalent=0
  Voltage Measurement : spsVoltageMeasurementLib/Voltage Measurement  PhasorSimulation=off  OutputType=Complex  PSBequivalent=0
  VDC+R : PMIOPort  Side=Right
  VDC-R : PMIOPort  Port=2  Side=Right
  VDC+L : PMIOPort  Port=3  Side=Left
  VDC-L : PMIOPort  Port=4  Side=Left
  I : Outport
  V : Outport  Port=2
  wires:
  Current Measurement/1 -> I/1
  Voltage Measurement/1 -> V/1
  connections:
  Current Measurement/LConn1 -- Voltage Measurement/LConn1 -- VDC+L/RConn1
  Current Measurement/RConn1 -- VDC+R/RConn1
  Voltage Measurement/LConn2 -- VDC-R/RConn1 -- VDC-L/RConn1

== system myLibrary/GFOL ==
  Constant5 : Constant  Value=[ 2/3 1/3; -1/3 1/3 ; -1/3 -2/3]
  Control : Subsystem
      settings: PortSchema="{\"entries\":[{\"content\":{\"sides\":[{\"content\":{},\"type\":\"ConnectorPlacement.EquallySpacedRectSide\",\"uuid\":\"681c0b5f-022d-4b6d-8fe2-73940743a76e\"},{\"content\":{\"side\":\"RIGHT\"},\"type\":\"ConnectorPlacement.EquallySpacedRectSide\",\"uuid\":\"e9b400c8-e13f-4caf-91a1-f348979675fd\"},{\"content\":{\"connectorIds\":[\"In1\",\"Out1\"],\"side\":\"TOP\"},\"type\":\"ConnectorPlacement.EquallySpacedRectSide\",\"uuid\":\"348007cb-ce67-4c45-ad7b-36ba89db6185\"},{\"content\":{\"connectorIds\":[\"In2\",\"In3\"],\"side\":\"BOTTOM\"},\"type\":\"ConnectorPlacement.EquallySpacedRectSide\",\"uuid\":\"fd6a847a-5d69-44cd-a0d1-495126761350\"}]},\"type\":\"ConnectorPlacement.EquallySpacedConnector\",\"uuid\":\"d16b8cae-5ced-4c76-a87e-983e154fb48f\"}],\"packageUris\":[\"http://schema.mathworks.com/mf0/Connector/R2020b\"],\"version\":\"1.0\"}"
  Current Measurement20 : spsCurrentMeasurementLib/Current Measurement  PhasorSimulation=off  OutputType=Complex  PSBequivalent=0
  Current Measurement21 : spsCurrentMeasurementLib/Current Measurement  PhasorSimulation=off  OutputType=Complex  PSBequivalent=0
  Current Measurement25 : spsCurrentMeasurementLib/Current Measurement  PhasorSimulation=off  OutputType=Complex  PSBequivalent=0
  Electrical : Subsystem
  Ig_l2g : Gain  Gain=1/T_VSC.Ibpu_l2g
  Is_l2g : Gain  Gain=1/T_VSC.Ibpu_l2g
  Mux10 : Mux  Inputs=2
  Mux4 : Mux  Inputs=3
  Product4 : Product  Multiplication=Matrix(*)
  Scope : Scope  NumInputPorts=3
  Series RLC Branch1 : spsSeriesRLCBranchLib/Series RLC Branch  LConnTagsString=__new0  RConnTagsString=__new0  BranchType=RL  Resistance=initVSC.Rtr  Inductance=initVSC.Ltr  SetiL0=off  InitialCurrent=initVSC.Iga  Capacitance=P.C  Setx0=on  InitialVoltage=P.C  Measurements=None
  Series RLC Branch10 : spsSeriesRLCBranchLib/Series RLC Branch  LConnTagsString=__new0  RConnTagsString=__new0  BranchType=R  Resistance=initVSC.Rac  Inductance=Lf  SetiL0=off  InitialCurrent=0  Capacitance=Cac_n1  Setx0=on  InitialVoltage=vcini_n1  Measurements=None
  Series RLC Branch2 : spsSeriesRLCBranchLib/Series RLC Branch  LConnTagsString=__new0  RConnTagsString=__new0  BranchType=RL  Resistance=initVSC.Rtr  Inductance=initVSC.Ltr  SetiL0=on  InitialCurrent=initVSC.Igb  Capacitance=P.C  Setx0=on  InitialVoltage=P.C  Measurements=None
  Series RLC Branch3 : spsSeriesRLCBranchLib/Series RLC Branch  LConnTagsString=__new0  RConnTagsString=__new0  BranchType=RL  Resistance=initVSC.Rtr  Inductance=initVSC.Ltr  SetiL0=on  InitialCurrent=initVSC.Igc  Capacitance=P.C  Setx0=on  InitialVoltage=P.C  Measurements=None
  Series RLC Branch4 : spsSeriesRLCBranchLib/Series RLC Branch  LConnTagsString=__new0  RConnTagsString=__new0  BranchType=C  Resistance=Rac_n1  Inductance=Lf  SetiL0=off  InitialCurrent=0  Capacitance=initVSC.Cac  Setx0=on  InitialVoltage=initVSC.Ucap_b  Measurements=None
  Series RLC Branch5 : spsSeriesRLCBranchLib/Series RLC Branch  LConnTagsString=__new0  RConnTagsString=__new0  BranchType=C  Resistance=Rac_n1  Inductance=Lf  SetiL0=off  InitialCurrent=0  Capacitance=initVSC.Cac  Setx0=on  InitialVoltage=initVSC.Ucap_a  Measurements=None
  Series RLC Branch6 : spsSeriesRLCBranchLib/Series RLC Branch  LConnTagsString=__new0  RConnTagsString=__new0  BranchType=R  Resistance=initVSC.Rac  Inductance=Lf  SetiL0=off  InitialCurrent=0  Capacitance=Cac_n1  Setx0=on  InitialVoltage=vcini_n1  Measurements=None
  Series RLC Branch8 : spsSeriesRLCBranchLib/Series RLC Branch  LConnTagsString=__new0  RConnTagsString=__new0  BranchType=R  Resistance=initVSC.Rac  Inductance=Lf  SetiL0=off  InitialCurrent=0  Capacitance=Cac_n1  Setx0=on  InitialVoltage=vcini_n1  Measurements=None
  Series RLC Branch9 : spsSeriesRLCBranchLib/Series RLC Branch  LConnTagsString=__new0  RConnTagsString=__new0  BranchType=C  Resistance=Rac_n1  Inductance=Lf  SetiL0=off  InitialCurrent=0  Capacitance=initVSC.Cac  Setx0=on  InitialVoltage=initVSC.Ucap_c  Measurements=None
  U_g2l : Gain  Gain=1/T_VSC.Vbpu_l2g
  Vdiff_l2g : Gain  Gain=T_VSC.Vbpu_l2g
  Voltage Measurement{,1..4} (5 alike) : spsVoltageMeasurementLib/Voltage Measurement  PhasorSimulation=off  OutputType=Complex  PSBequivalent=0
  VA : PMIOPort  Side=Right
  VB : PMIOPort  Port=2  Side=Right
  VC : PMIOPort  Port=3  Side=Right
  wires:
  Voltage Measurement4/1 -> Scope/3
  Voltage Measurement2/1 -> Scope/1
  Voltage Measurement3/1 -> Scope/2
  Ig_l2g/1 -> Control/1(ig_abc)
  Current Measurement25/1 -> Mux4/3
  Mux4/1 -> Ig_l2g/1
  Current Measurement21/1 -> Mux4/1
  Current Measurement20/1 -> Mux4/2
  U_g2l/1 -> Control/2(U)
  Is_l2g/1 -> Control/3(Iss)
  Vdiff_l2g/1 -> Electrical/1(Vdiff)
  Electrical/1(Is) -> Is_l2g/1
  Control/1(Vdiff_abc) -> Vdiff_l2g/1
  Product4/1 -> U_g2l/1
  Voltage Measurement/1 -> Mux10/1
  Mux10/1 -> Product4/2
  Constant5/1 -> Product4/1
  Voltage Measurement1/1 -> Mux10/2
  connections:
  Series RLC Branch6/RConn1 -- Series RLC Branch8/RConn1 -- Series RLC Branch10/RConn1
  Series RLC Branch9/RConn1 -- Series RLC Branch10/LConn1 -- Voltage Measurement4/LConn2
  Series RLC Branch8/LConn1 -- Series RLC Branch4/RConn1 -- Voltage Measurement3/LConn2
  Series RLC Branch5/RConn1 -- Series RLC Branch6/LConn1 -- Voltage Measurement2/LConn2
  Series RLC Branch3/RConn1 -- Current Measurement25/LConn1
  Series RLC Branch2/RConn1 -- Current Measurement20/LConn1
  Series RLC Branch1/RConn1 -- Current Measurement21/LConn1
  Current Measurement25/RConn1 -- VC/RConn1
  Electrical/LConn2 -- Voltage Measurement/LConn2 -- Series RLC Branch2/LConn1 -- Voltage Measurement3/LConn1 -- Series RLC Branch4/LConn1 -- Voltage Measurement1/LConn1
  VA/RConn1 -- Current Measurement21/RConn1
  Electrical/LConn3 -- Series RLC Branch3/LConn1 -- Voltage Measurement4/LConn1 -- Series RLC Branch9/LConn1 -- Voltage Measurement1/LConn2
  Electrical/LConn1 -- Voltage Measurement/LConn1 -- Voltage Measurement2/LConn1 -- Series RLC Branch5/LConn1 -- Series RLC Branch1/LConn1
  VB/RConn1 -- Current Measurement20/RConn1

== system myLibrary/GFOL_RL ==
  Constant5 : Constant  Value=[ 2/3 1/3; -1/3 1/3 ; -1/3 -2/3]
  Control : Subsystem
      settings: PortSchema="{\"entries\":[{\"content\":{\"sides\":[{\"content\":{\"connectorIds\":[]},\"type\":\"ConnectorPlacement.EquallySpacedRectSide\",\"uuid\":\"681c0b5f-022d-4b6d-8fe2-73940743a76e\"},{\"content\":{\"connectorIds\":[],\"side\":\"RIGHT\"},\"type\":\"ConnectorPlacement.EquallySpacedRectSide\",\"uuid\":\"e9b400c8-e13f-4caf-91a1-f348979675fd\"},{\"content\":{\"connectorIds\":[\"Out1\"],\"side\":\"TOP\"},\"type\":\"ConnectorPlacement.EquallySpacedRectSide\",\"uuid\":\"348007cb-ce67-4c45-ad7b-36ba89db6185\"},{\"content\":{\"connectorIds\":[\"In1\",\"In2\"],\"side\":\"BOTTOM\"},\"type\":\"ConnectorPlacement.EquallySpacedRectSide\",\"uuid\":\"fd6a847a-5d69-44cd-a0d1-495126761350\"}]},\"type\":\"ConnectorPlacement.EquallySpacedConnector\",\"uuid\":\"d16b8cae-5ced-4c76-a87e-983e154fb48f\"}],\"packageUris\":[\"http://schema.mathworks.com/mf0/Connector/R2020b\"],\"version\":\"1.0\"}"
  Electrical : Subsystem
  Is_l2g : Gain  Gain=1/T_VSC.Ibpu_l2g
  Mux10 : Mux  Inputs=2
  Product4 : Product  Multiplication=Matrix(*)
  Series RLC Branch1 : spsSeriesRLCBranchLib/Series RLC Branch  LConnTagsString=__new0  RConnTagsString=__new0  BranchType=RL  Resistance=initVSC.Rtr  Inductance=initVSC.Ltr  SetiL0=off  InitialCurrent=initVSC.Iga  Capacitance=P.C  Setx0=on  InitialVoltage=P.C  Measurements=None
  Series RLC Branch2 : spsSeriesRLCBranchLib/Series RLC Branch  LConnTagsString=__new0  RConnTagsString=__new0  BranchType=RL  Resistance=initVSC.Rtr  Inductance=initVSC.Ltr  SetiL0=on  InitialCurrent=initVSC.Igb  Capacitance=P.C  Setx0=on  InitialVoltage=P.C  Measurements=None
  Series RLC Branch3 : spsSeriesRLCBranchLib/Series RLC Branch  LConnTagsString=__new0  RConnTagsString=__new0  BranchType=RL  Resistance=initVSC.Rtr  Inductance=initVSC.Ltr  SetiL0=on  InitialCurrent=initVSC.Igc  Capacitance=P.C  Setx0=on  InitialVoltage=P.C  Measurements=None
  U_g2l : Gain  Gain=1/T_VSC.Vbpu_l2g
  Vdiff_l2g : Gain  Gain=T_VSC.Vbpu_l2g
  Voltage Measurement : spsVoltageMeasurementLib/Voltage Measurement  PhasorSimulation=off  OutputType=Complex  PSBequivalent=0
  Voltage Measurement1 : spsVoltageMeasurementLib/Voltage Measurement  PhasorSimulation=off  OutputType=Complex  PSBequivalent=0
  VA : PMIOPort  Side=Right
  VB : PMIOPort  Port=2  Side=Right
  VC : PMIOPort  Port=3  Side=Right
  wires:
  U_g2l/1 -> Control/1(U)
  Is_l2g/1 -> Control/2(Iss)
  Vdiff_l2g/1 -> Electrical/1(Vdiff)
  Electrical/1(Is) -> Is_l2g/1
  Control/1(Vdiff_abc) -> Vdiff_l2g/1
  Product4/1 -> U_g2l/1
  Voltage Measurement/1 -> Mux10/1
  Mux10/1 -> Product4/2
  Constant5/1 -> Product4/1
  Voltage Measurement1/1 -> Mux10/2
  connections:
  Series RLC Branch3/RConn1 -- VC/RConn1
  Voltage Measurement/LConn2 -- Series RLC Branch2/LConn1 -- Voltage Measurement1/LConn1 -- Electrical/LConn2
  VA/RConn1 -- Series RLC Branch1/RConn1
  Electrical/LConn3 -- Series RLC Branch3/LConn1 -- Voltage Measurement1/LConn2
  Series RLC Branch1/LConn1 -- Voltage Measurement/LConn1 -- Electrical/LConn1
  VB/RConn1 -- Series RLC Branch2/RConn1

== system myLibrary/GFOR ==
  Constant5 : Constant  Value=[ 2/3 1/3; -1/3 1/3 ; -1/3 -2/3]
  Control : Subsystem
      settings: PortSchema="{\"entries\":[{\"content\":{\"sides\":[{\"content\":{},\"type\":\"ConnectorPlacement.EquallySpacedRectSide\",\"uuid\":\"681c0b5f-022d-4b6d-8fe2-73940743a76e\"},{\"content\":{\"side\":\"RIGHT\"},\"type\":\"ConnectorPlacement.EquallySpacedRectSide\",\"uuid\":\"e9b400c8-e13f-4caf-91a1-f348979675fd\"},{\"content\":{\"connectorIds\":[\"In1\",\"Out1\"],\"side\":\"TOP\"},\"type\":\"ConnectorPlacement.EquallySpacedRectSide\",\"uuid\":\"348007cb-ce67-4c45-ad7b-36ba89db6185\"},{\"content\":{\"connectorIds\":[\"In2\",\"In3\"],\"side\":\"BOTTOM\"},\"type\":\"ConnectorPlacement.EquallySpacedRectSide\",\"uuid\":\"fd6a847a-5d69-44cd-a0d1-495126761350\"}]},\"type\":\"ConnectorPlacement.EquallySpacedConnector\",\"uuid\":\"d16b8cae-5ced-4c76-a87e-983e154fb48f\"}],\"packageUris\":[\"http://schema.mathworks.com/mf0/Connector/R2020b\"],\"version\":\"1.0\"}"
  Current Measurement20 : spsCurrentMeasurementLib/Current Measurement  PhasorSimulation=off  OutputType=Complex  PSBequivalent=0
  Current Measurement21 : spsCurrentMeasurementLib/Current Measurement  PhasorSimulation=off  OutputType=Complex  PSBequivalent=0
  Current Measurement25 : spsCurrentMeasurementLib/Current Measurement  PhasorSimulation=off  OutputType=Complex  PSBequivalent=0
  Electrical : Subsystem
  Ig_l2g : Gain  Gain=1/T_VSC.Ibpu_l2g
  Is_l2g : Gain  Gain=1/T_VSC.Ibpu_l2g
  Mux10 : Mux  Inputs=2
  Mux4 : Mux  Inputs=3
  Product4 : Product  Multiplication=Matrix(*)
  Scope : Scope  NumInputPorts=3
  Series RLC Branch1 : spsSeriesRLCBranchLib/Series RLC Branch  LConnTagsString=__new0  RConnTagsString=__new0  BranchType=RL  Resistance=initVSC.Rtr  Inductance=initVSC.Ltr  SetiL0=off  InitialCurrent=initVSC.Iga  Capacitance=P.C  Setx0=on  InitialVoltage=P.C  Measurements=None
  Series RLC Branch10 : spsSeriesRLCBranchLib/Series RLC Branch  LConnTagsString=__new0  RConnTagsString=__new0  BranchType=R  Resistance=initVSC.Rac  Inductance=Lf  SetiL0=off  InitialCurrent=0  Capacitance=Cac_n1  Setx0=on  InitialVoltage=vcini_n1  Measurements=None
  Series RLC Branch2 : spsSeriesRLCBranchLib/Series RLC Branch  LConnTagsString=__new0  RConnTagsString=__new0  BranchType=RL  Resistance=initVSC.Rtr  Inductance=initVSC.Ltr  SetiL0=on  InitialCurrent=initVSC.Igb  Capacitance=P.C  Setx0=on  InitialVoltage=P.C  Measurements=None
  Series RLC Branch3 : spsSeriesRLCBranchLib/Series RLC Branch  LConnTagsString=__new0  RConnTagsString=__new0  BranchType=RL  Resistance=initVSC.Rtr  Inductance=initVSC.Ltr  SetiL0=on  InitialCurrent=initVSC.Igc  Capacitance=P.C  Setx0=on  InitialVoltage=P.C  Measurements=None
  Series RLC Branch4 : spsSeriesRLCBranchLib/Series RLC Branch  LConnTagsString=__new0  RConnTagsString=__new0  BranchType=C  Resistance=Rac_n1  Inductance=Lf  SetiL0=off  InitialCurrent=0  Capacitance=initVSC.Cac  Setx0=on  InitialVoltage=initVSC.Ucap_b  Measurements=None
  Series RLC Branch5 : spsSeriesRLCBranchLib/Series RLC Branch  LConnTagsString=__new0  RConnTagsString=__new0  BranchType=C  Resistance=Rac_n1  Inductance=Lf  SetiL0=off  InitialCurrent=0  Capacitance=initVSC.Cac  Setx0=on  InitialVoltage=initVSC.Ucap_a  Measurements=None
  Series RLC Branch6 : spsSeriesRLCBranchLib/Series RLC Branch  LConnTagsString=__new0  RConnTagsString=__new0  BranchType=R  Resistance=initVSC.Rac  Inductance=Lf  SetiL0=off  InitialCurrent=0  Capacitance=Cac_n1  Setx0=on  InitialVoltage=vcini_n1  Measurements=None
  Series RLC Branch8 : spsSeriesRLCBranchLib/Series RLC Branch  LConnTagsString=__new0  RConnTagsString=__new0  BranchType=R  Resistance=initVSC.Rac  Inductance=Lf  SetiL0=off  InitialCurrent=0  Capacitance=Cac_n1  Setx0=on  InitialVoltage=vcini_n1  Measurements=None
  Series RLC Branch9 : spsSeriesRLCBranchLib/Series RLC Branch  LConnTagsString=__new0  RConnTagsString=__new0  BranchType=C  Resistance=Rac_n1  Inductance=Lf  SetiL0=off  InitialCurrent=0  Capacitance=initVSC.Cac  Setx0=on  InitialVoltage=initVSC.Ucap_c  Measurements=None
  U_g2l : Gain  Gain=1/T_VSC.Vbpu_l2g
  Vdiff_l2g : Gain  Gain=T_VSC.Vbpu_l2g
  Voltage Measurement{,1..4} (5 alike) : spsVoltageMeasurementLib/Voltage Measurement  PhasorSimulation=off  OutputType=Complex  PSBequivalent=0
  VA : PMIOPort  Side=Right
  VB : PMIOPort  Port=2  Side=Right
  VC : PMIOPort  Port=3  Side=Right
  wires:
  U_g2l/1 -> Control/2(Uabc)
  Vdiff_l2g/1 -> Electrical/1(Vdiff)
  Ig_l2g/1 -> Control/1(ig_abc)
  Is_l2g/1 -> Control/3(Iss)
  Voltage Measurement4/1 -> Scope/3
  Voltage Measurement3/1 -> Scope/2
  Voltage Measurement2/1 -> Scope/1
  Voltage Measurement1/1 -> Mux10/2
  Constant5/1 -> Product4/1
  Mux10/1 -> Product4/2
  Voltage Measurement/1 -> Mux10/1
  Product4/1 -> U_g2l/1
  Control/1(Vdiff_abc) -> Vdiff_l2g/1
  Electrical/1(Is) -> Is_l2g/1
  Current Measurement21/1 -> Mux4/1
  Mux4/1 -> Ig_l2g/1
  Current Measurement25/1 -> Mux4/3
  Current Measurement20/1 -> Mux4/2
  connections:
  Series RLC Branch1/LConn1 -- Series RLC Branch5/LConn1 -- Voltage Measurement2/LConn1 -- Voltage Measurement/LConn1 -- Electrical/LConn1
  Series RLC Branch2/LConn1 -- Series RLC Branch4/LConn1 -- Voltage Measurement3/LConn1 -- Voltage Measurement1/LConn1 -- Electrical/LConn2 -- Voltage Measurement/LConn2
  Series RLC Branch3/LConn1 -- Series RLC Branch9/LConn1 -- Voltage Measurement4/LConn1 -- Voltage Measurement1/LConn2 -- Electrical/LConn3
  Current Measurement21/RConn1 -- VA/RConn1
  Current Measurement25/RConn1 -- VC/RConn1
  VB/RConn1 -- Current Measurement20/RConn1
  Current Measurement25/LConn1 -- Series RLC Branch3/RConn1
  Series RLC Branch2/RConn1 -- Current Measurement20/LConn1
  Series RLC Branch1/RConn1 -- Current Measurement21/LConn1
  Series RLC Branch6/RConn1 -- Series RLC Branch10/RConn1 -- Series RLC Branch8/RConn1
  Series RLC Branch5/RConn1 -- Voltage Measurement2/LConn2 -- Series RLC Branch6/LConn1
  Series RLC Branch9/RConn1 -- Voltage Measurement4/LConn2 -- Series RLC Branch10/LConn1
  Series RLC Branch8/LConn1 -- Voltage Measurement3/LConn2 -- Series RLC Branch4/RConn1
